simulink model "t1"  (Simulink 7.5)
settings: Solver=ode3  StartTime=0.0  StopTime=20  RelTol=1e-3
undefined symbols (not defined in the file): DiscIntNeverNeededParam
settings Model: Creator=Dranik_win  LastModifiedBy=Dranik_win

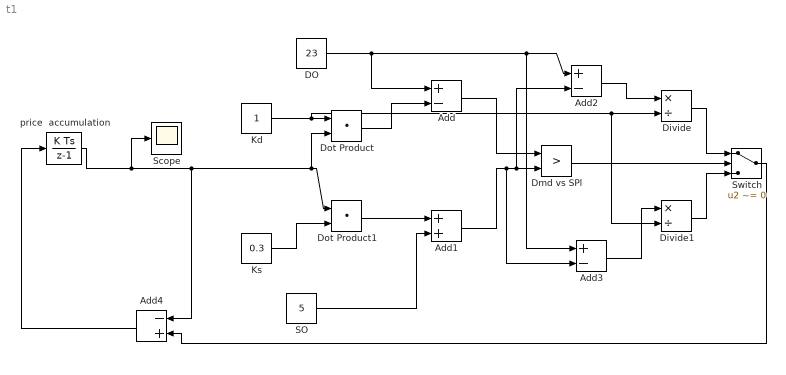
== system t1 ==
  Add : Sum  Inputs=+-  OutDataType=fixdt(1, 16)  OutScaling=2^-10
  Add1 : Sum  OutDataType=fixdt(1, 16)  OutScaling=2^-10
  Add2 : Sum  Inputs=+-  OutDataType=fixdt(1, 16)  OutScaling=2^-10
  Add3 : Sum  Inputs=+-  OutDataType=fixdt(1, 16)  OutScaling=2^-10
  Add4 : Sum  Inputs=-+  OutDataType=fixdt(1, 16)  OutScaling=2^-10
  DO : Constant  Value=23  OutDataType=fixdt(1, 16)  OutScaling=2^0
  Divide : Product  Inputs=*/  OutDataType=fixdt(1, 16)  OutScaling=2^-10
  Divide1 : Product  Inputs=*/  OutDataType=fixdt(1, 16)  OutScaling=2^-10
  Dmd vs SPl : RelationalOperator  Operator=>  LogicOutDataTypeMode=boolean  LogicDataType=fixdt(0, 8)  OutDataTypeStr=boolean
  Dot Product : DotProduct  OutDataType=fixdt(1, 16)  OutScaling=2^-10  InputSameDT=on  OutDataTypeStr=Inherit: Inherit via internal rule
  Dot Product1 : DotProduct  OutDataType=fixdt(1, 16)  OutScaling=2^-10  InputSameDT=on  OutDataTypeStr=Inherit: Inherit via internal rule
  Kd : Constant  OutDataType=fixdt(1, 16)  OutScaling=2^0
  Ks : Constant  Value=0.3  OutDataType=fixdt(1, 16)  OutScaling=2^0
  SO : Constant  Value=5  OutDataType=fixdt(1, 16)  OutScaling=2^0
  Scope : Scope
  Switch : Switch  Criteria=u2 ~= 0  OutDataType=fixdt(1, 16)  OutScaling=2^0
  price  accumulation : DiscreteIntegrator  InitialCondition=10  OutDataType=fixdt(1, 16)  OutScaling=2^0  ICPrevOutput=DiscIntNeverNeededParam  ICPrevScaledInput=DiscIntNeverNeededParam
  wires:
  Kd/1 -> Dot Product/1, Divide/2, Divide1/2
  price  accumulation/1 -> Dot Product/2, Dot Product1/1, Add4/1, Scope/1
  DO/1 -> Add/1, Add2/1, Add3/1
  Dot Product/1 -> Add/2
  Ks/1 -> Dot Product1/2
  Dot Product1/1 -> Add1/1
  SO/1 -> Add1/2
  Add1/1 -> Dmd vs SPl/2, Add2/2, Add3/2
  Add/1 -> Dmd vs SPl/1
  Dmd vs SPl/1 -> Switch/2
  Add2/1 -> Divide/1
  Divide/1 -> Switch/1
  Add3/1 -> Divide1/1
  Divide1/1 -> Switch/3
  Switch/1 -> Add4/2
  Add4/1 -> price  accumulation/1
